simulink model "quad_CAD_asgsm"  (R2024a)
settings: Solver=ode4  StartTime=0.0  StopTime=60  FixedStep=0.01  RelTol=1e-3
undefined symbols (not defined in the file): F, Light, MIL, smiData, X, Y, Z
libraries: sm_lib x221, nesl_utility x22, dspobslib x9, sharedtransform x6, simulink x3, aerolibutil x2, matrix_library x1, sharedutil x1, robotcorelib x1, aerolibwind2 x1
(part 1 of 7)
Description:
  | Adaptive Single-Gain Sliding Mode Controller for a quadrotor modelled in
  | Simscape Multibody
settings Model: Creator=adanm  LastModifiedBy=adanm

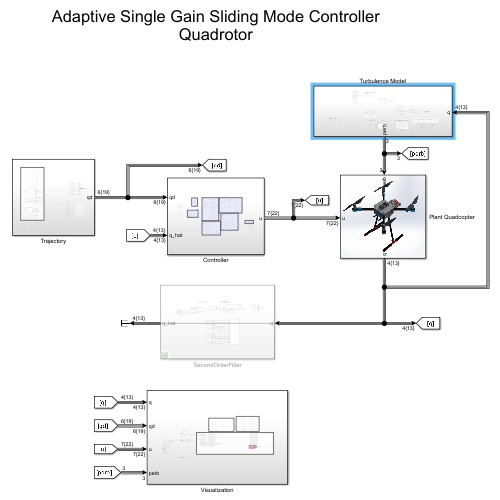
[thumbnail: Simulink's stored preview of the top-level diagram]
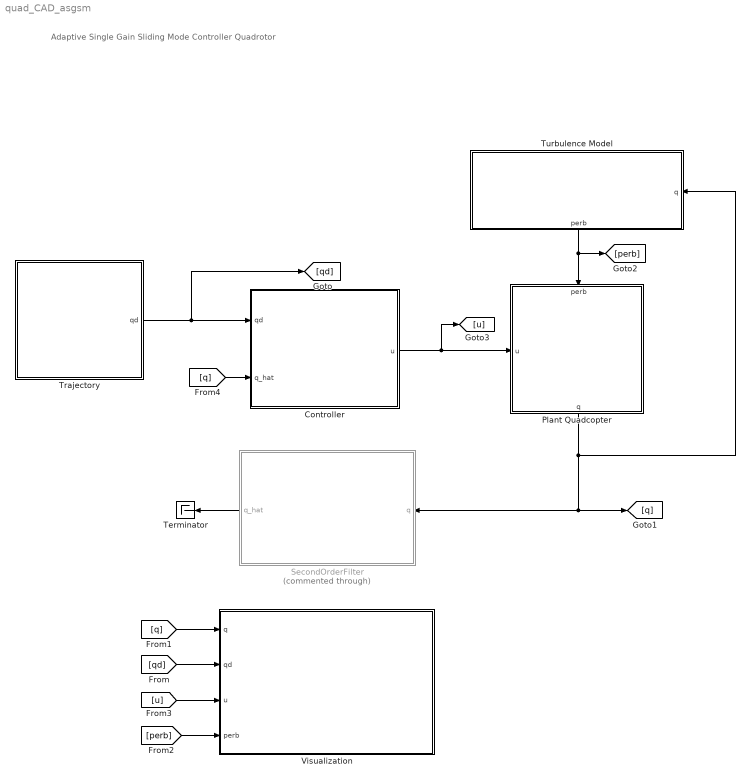
== system quad_CAD_asgsm ==
  note: Adaptive Single Gain Sliding Mode Controller
      | Quadrotor
  Controller : Subsystem
  Plant Quadcopter : Subsystem
      settings: PortSchema="{\"entries\":[{\"content\":{\"sides\":[{\"content\":{\"connectorIds\":[\"In1\"]},\"type\":\"ConnectorPlacement.EquallySpacedRectSide\",\"uuid\":\"f949eb9b-1537-4457-8173-53f8756fded2\"},{\"content\":{\"side\":\"RIGHT\"},\"type\":\"ConnectorPlacement.EquallySpacedRectSide\",\"uuid\":\"4fbfc7d4-94f2-46a4-b9fc-ef834e77a9ed\"},{\"content\":{\"connectorIds\":[\"In2\"],\"side\":\"TOP\"},\"type\":\"ConnectorPlacement.EquallySpacedRectSide\",\"uuid\":\"37f6ffd5-491e-413a-8e1b-4483447938c5\"},{\"content\":{\"connectorIds\":[\"Out1\"],\"side\":\"BOTTOM\"},\"type\":\"ConnectorPlacement.EquallySpacedRectSide\",\"uuid\":\"c1c386c7-2f11-4e96-8840-db3d41072bec\"}]},\"type\":\"ConnectorPlacement.EquallySpacedConnector\",\"uuid\":\"4c6ce227-67e5-4051-af2d-189fa0d9d7e1\"}],\"packageUris\":[\"http://schema.mathworks.com/mf0/Connector/R2020b\"],\"version\":\"1.0\"}"
      mask Display: image('quadRender.png');
  SecondOrderFilter : Subsystem  Commented=through
      settings: PortSchema="{\"entries\":[{\"content\":{\"sides\":[{\"content\":{\"connectorIds\":[\"Out1\"]},\"type\":\"ConnectorPlacement.EquallySpacedRectSide\",\"uuid\":\"b4c8c2cb-3651-490a-ad01-89b97c3933b2\"},{\"content\":{\"connectorIds\":[\"In1\"],\"side\":\"RIGHT\"},\"type\":\"ConnectorPlacement.EquallySpacedRectSide\",\"uuid\":\"f3956ee2-2beb-41a9-b697-53efa6c7f661\"},{\"content\":{\"side\":\"TOP\"},\"type\":\"ConnectorPlacement.EquallySpacedRectSide\",\"uuid\":\"338fc46d-6a44-4c7a-9eb5-4ab91a191b04\"}]},\"type\":\"ConnectorPlacement.EquallySpacedConnector\",\"uuid\":\"d4e003fa-30a1-40f4-b71f-e0999cd1b71b\"}],\"packageUris\":[\"http://schema.mathworks.com/mf0/Connector/R2020b\"],\"version\":\"1.0\"}"
  Terminator : Terminator
  Trajectory : Subsystem
  Turbulence Model : Subsystem
      settings: PortSchema="{\"entries\":[{\"content\":{\"sides\":[{\"content\":{},\"type\":\"ConnectorPlacement.EquallySpacedRectSide\",\"uuid\":\"f78b09a1-2be7-4ada-a431-40e3e9754158\"},{\"content\":{\"connectorIds\":[\"In1\"],\"side\":\"RIGHT\"},\"type\":\"ConnectorPlacement.EquallySpacedRectSide\",\"uuid\":\"90af6136-accc-442b-9679-ef2510f8cfdd\"},{\"content\":{\"side\":\"TOP\"},\"type\":\"ConnectorPlacement.EquallySpacedRectSide\",\"uuid\":\"ed3143b1-02fd-44b4-8f22-c95c41bbcf7f\"},{\"content\":{\"connectorIds\":[\"Out1\"],\"side\":\"BOTTOM\"},\"type\":\"ConnectorPlacement.EquallySpacedRectSide\",\"uuid\":\"715dd93d-905b-40a3-aeb3-61c6c8d9767d\"}]},\"type\":\"ConnectorPlacement.EquallySpacedConnector\",\"uuid\":\"95dc4bc2-a941-4378-8d0a-e3a54b47d1ac\"}],\"packageUris\":[\"http://schema.mathworks.com/mf0/Connector/R2020b\"],\"version\":\"1.0\"}"
  Visualization : Subsystem
  wires:
  Turbulence Model/1(perb) -> [perb], Plant Quadcopter/2(perb)
  Plant Quadcopter/1(q) -> Turbulence Model/1(q), SecondOrderFilter/1(q), [q]
  Trajectory/1(qd) -> [qd], Controller/1(qd)
  SecondOrderFilter/1(q_hat) -> Terminator/1
  Controller/1(u) -> [u], Plant Quadcopter/1(u)
  [qd] -> Visualization/2(qd)
  [q] -> Visualization/1(q)
  [perb] -> Visualization/4(perb)
  [u] -> Visualization/3(u)
  [q] -> Controller/2(q_hat)

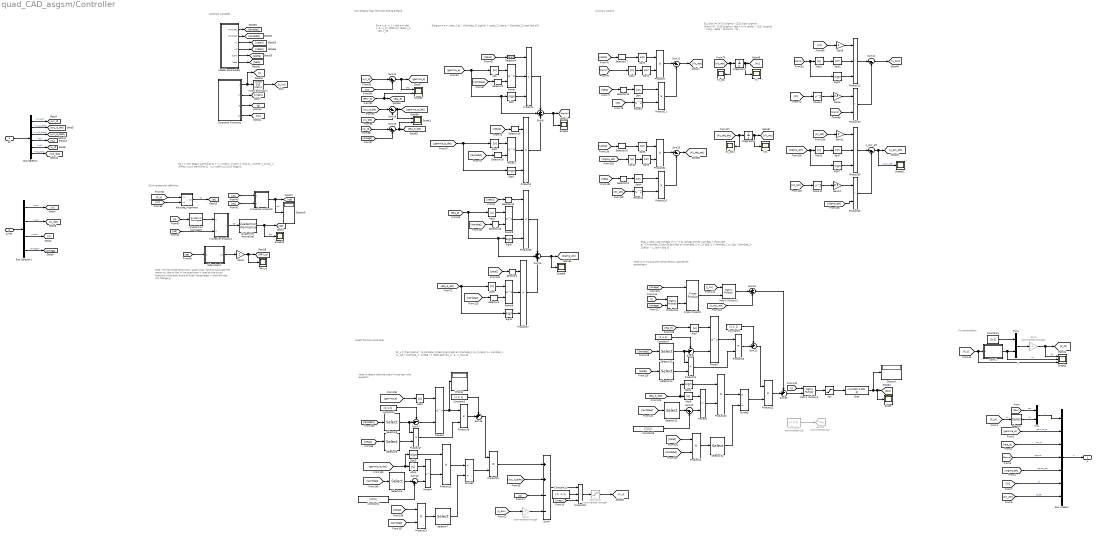
== system quad_CAD_asgsm/Controller ==
  note: $q_t = \pm \Bigg [ \sqrt{\frac{1 + n_u \cdot n_z}{2}} + \frac{n_u \times n_z}{||n_u \times n_z||} \sqrt{\frac{1 - n_u \cdot n_z}{2}} \Bigg ]$
  note: Note: It seems that the mass if missing in
      | the equation.
  note: Note: It is missing the Inertia Tensor outside
      | the parenthesis
  note: $F_u = \frac{|\dot e|^{2-\lambda_2}\text{sign}(\dot e)}{\lambda_2 \xi_2} \Big (1 + \lambda_1 \xi_1|e|^{\lambda_1 - 1}\Big ) + \ddot \gamma_d - g - u_{aux}$
  note: ANSFT Position Controller
  note: $e = x_d - x_1 \\ \dot e = \dot x_d - x_2 \\ \ddot e = \ddot x_d - \dot x_2$
  note: $\sigma = e + \zeta_1 |e| ^{\lambda_1} sign(e) + \zeta_2 | \dot e| ^{\lambda_2} sign(\dot e)$
  note: $u_{aux}=-2K(t) |\sigma|^{1/2} sign (\sigma) - \frac{K(t)^2}{2}\sigma \\ \dot K(t) = \alpha ^{1/2} |\sigma| ^{1/2} - \beta ^{1/2}K(t)^2$
  note: Non-Singular Fast Terminal Sliding Surface
  note: $\tau = \Big [ \dot \omega_d + J^{-1} \omega \times J \omega + \frac{|\dot e|^{2-\lambda_2}\text{sign}(\dot e)}{\lambda_2 \xi_2} \Big (1 + \lambda_1 \xi_1|e|^{\lambda_1 - 1}\Big ) - u_{aux} \Big ]$
  note: Auxiliary Control
  note: Constant variables
  note: Note : For the tilted Hexa-rotor I guess that I
      | have to calculate the vector nz, due to that in the
      | quad-rotor it used as the thrust direction in the body
      | frame of itself. Nonetheless in the FAH that will change ig
  note: Error quaternion definition
  note: Fu manipulation
  qd : Inport
  q_hat : Inport  Port=2
  ASGSM parameters : MATLAB Function  TreatAsAtomicUnit=on
  Abs{,1..11} (12 alike) : Abs  SaturateOnIntegerOverflow=off
  Attitude_Alignment : Subsystem
  Bias : Bias  Bias=[0.002; 0.025; 0]  SaturateOnIntegerOverflow=off
  Bus Creator : BusCreator  Inputs=7
  Bus Selector : BusSelector  OutputSignals=xyz_d,xyz_d_dot,xyz_d_ddot,qz,wd,wd_dot
  Bus Selector1 : BusSelector  OutputSignals=pos,vel,quat,omega
  Constant1 : Constant  Value=[0; 0]
  Constant11 : Constant  Value=[-1; -1; 1]
  Constant{3,5,7,9} (4 alike) : Constant  Value=[1; 1; 1]
  Constant4 : Constant  Value=[2;2;2]
  Constant6 : Constant  Commented=on  Value=[0; 0; 0]
  Constant8 : Constant  Value=[2;2;2]
  Constants Functions : MATLAB Function  TreatAsAtomicUnit=on
  Cross Product1 : matrix_library/Cross Product
  Display : Display
  Display1 : Display
  Display6 : Display
  Divide2 : Product  Inputs=*/
  Divide3 : Product  Inputs=*/
  Gain12 : Gain  Gain=2
  Gain13 : Gain  Gain=0.5
  Gain2 : Gain  Commented=through  Gain=-1
  Gain3 : Gain  Gain=2
  Gain4 : Gain  Commented=through  Gain=-1
  Gain6 : Gain  Gain=2
  Gain8 : Gain  Gain=0.5
  Goto59 : Goto  Commented=on  GotoTag=tau
  Integrator4 : Integrator  InitialCondition=[0;0;0]
  Integrator5 : Integrator  InitialCondition=[0;0;0]
  Invert 3x3 Matrix : aerolibutil/Invert  3x3 Matrix
  Kronecker product3 : Subsystem
  Kronecker product4 : Subsystem
  Kt : Scope
  Kt1 : Scope
  Kt_dot : Scope
  Kt_dot1 : Scope
  Matrix Multiply2 : Product  Multiplication=Matrix(*)
  Matrix Multiply5 : Product  Multiplication=Matrix(*)
  Mux : Mux  Inputs=2
  Mux1 : Mux  Inputs=2
  PRV_e : Scope
  Power{,1,4..9} (8 alike) : Math  Operator=pow
  Power{2..3,10..11} (4 alike) : Math  Operator=square
  Product{9..11,13..17,20..24,28..29,31} (16 alike) : Product
  Product{4,8,12,25..27,30} (7 alike) : Product  Inputs=3
  Product19 : Product  Multiplication=Matrix(*)
  Quaternion Conjugate : aerolibutil/Quaternion Conjugate
  Quaternion Normalize1 : sharedutil/Quaternion Normalize  aMode=aMode
  Saturation : Saturate  Commented=through  UpperLimit=4*10  LowerLimit=0
  Scope{,8..11} (5 alike) : Scope
  Scope1 : Scope  NumInputPorts=2
  Scope2 : Scope  NumInputPorts=3
  Scope3 : Scope  NumInputPorts=2
  Selector : Selector  InputPortWidth=3  IndexOptions=Index vector (dialog)  Indices=[3]  OutputSizes=1
  Selector{1,3,10..14,18,20..21} (10 alike) : Selector  InputPortWidth=6  IndexOptions=Index vector (dialog)  Indices=[4:6]  OutputSizes=1
  Selector{4..9,15..17,19} (10 alike) : Selector  InputPortWidth=6  IndexOptions=Index vector (dialog)  Indices=[1:3]  OutputSizes=1
  Sign{,1..7} (8 alike) : Signum
  Sqrt{,1..7} (8 alike) : Sqrt
  Subsystem1 : Subsystem
  Sum10 : Sum  Inputs=|-+
  Sum{11,14..16,25} (5 alike) : Sum  Inputs=|+-
  Sum12 : Sum  Inputs=|--
  Sum17 : Sum  Inputs=-+|
  Sum18 : Sum  Inputs=++|
  Sum19 : Sum  Inputs=++-
  Sum20 : Sum  Inputs=|-+
  Sum21 : Sum  Inputs=-+|
  Sum22 : Sum  Inputs=++|
  Sum23 : Sum  Inputs=++|
  Sum24 : Sum  Inputs=+++
  Sum6 : Sum  Inputs=++--
  Sum9 : Sum  Inputs=+++
  norm1 : MATLAB Function  TreatAsAtomicUnit=on
  tau : Saturate
  u_aux_att : Sum  Inputs=|--
  u : Outport
  wires:
  Sqrt5/1 -> Product31/1
  Sum14/1 -> Scope3/1, [gamma_e]  "des"
  Product28/1 -> u_aux_att/2
  u_aux_att/1 -> Scope11/1, [u_aux_att]  "u_aux_att"
  Sum12/1 -> [u_aux]
  Product29/1 -> Sum25/2
  Integrator4/1 -> Kt/1, [Kt]
  Selector19/1 -> Sqrt/1
  [J] -> Matrix Multiply5/1
  [sigma_att] -> Product28/2
  [g] -> Sum6/3
  Product22/1 -> Sum23/2
  Sum10/1 -> Power4/2
  Cross Product1/1 -> Matrix Multiply2/2
  Sqrt3/1 -> Product12/2
  Abs7/1 -> Power7/1
  Sum25/1 -> [Kt_dot_att]
  Selector20/1 -> Sqrt5/1
  [Kt_att] -> Gain12/1
  [lambda2] -> Selector3/1
  Selector18/1 -> Power8/2
  [omega] -> Cross Product1/1
  Sqrt7/1 -> Product30/2
  [xyz_d_ddot] -> Sum6/2
  Sum24/1 -> Scope8/1, [sigma_att]
  Product27/1 -> Sum24/3
  Selector7/1 -> Divide2/2
  Power10/1 -> Product29/2
  Sign6/1 -> Product27/3
  Sign/1 -> Product4/3
  Sum19/1 -> Sum23/1
  Abs11/1 -> Sqrt7/1
  [eta_e_dot] -> Abs9/1, Sign6/1
  Sum20/1 -> Power6/2
  Selector5/1 -> Power/2
  [gamma_e] -> Abs5/1
  [PRV_e] -> Scope3/2, [eta_e]
  [gamma_e] -> Sum9/2, Sign/1, Abs/1
  [eta_e] -> Sum24/2, Sign5/1, Abs8/1
  Power8/1 -> Product26/2
  Abs8/1 -> Power8/1
  Product26/1 -> Sum24/1
  Abs5/1 -> Power5/1
  Constant8/1 -> Sum20/2
  Selector3/1 -> Power9/2
  Selector17/1 -> Sqrt1/1
  Sum17/1 -> Power5/2
  Selector16/1 -> Power1/2
  Abs6/1 -> Power6/1
  [Kt_dot_att] -> Kt_dot1/1, Integrator5/1
  Constant9/1 -> Sum22/1
  [Kt_att] -> Power10/1
  Constant5/1 -> Sum18/1
  Sign7/1 -> Product30/3
  Selector9/1 -> Product17/2
  Sqrt4/1 -> Product29/1
  Constant11/1 -> Product25/2
  Abs1/1 -> Power1/1
  Product25/1 -> Saturation/1
  Selector21/1 -> Sqrt4/1
  Sum6/1 -> Product25/1
  [lambda1] -> Selector13/1
  Selector13/1 -> Product24/1, Sum21/2
  [Kt] -> Power2/1
  Power4/1 -> Product13/2
  Power7/1 -> Product23/1
  Selector12/1 -> Divide3/2
  [lambda2] -> Selector11/1
  Constant3/1 -> Sum17/1
  Sum11/1 -> [Kt_dot]
  Sign4/1 -> Product20/1
  Product23/1 -> Sum22/2
  [lambda2] -> Product21/2
  Product21/1 -> Selector12/1
  Constant7/1 -> Sum21/1
  Power6/1 -> Product20/2
  Selector14/1 -> Product24/2
  [zeta2] -> Product21/1
  Power1/1 -> Product8/2
  [J_inv] -> Matrix Multiply2/1
  Product15/1 -> Sum6/1
  Matrix Multiply5/1 -> tau/1
  Product17/1 -> Product16/2
  Product16/1 -> Sum18/2
  Product20/1 -> Divide3/1
  Power9/1 -> Product27/2
  [w_d] -> Sum16/1
  Abs3/1 -> Sqrt3/1
  Selector8/1 -> Product17/1, Sum17/2
  Gain4/1 -> Sum6/4
  Product14/1 -> Selector7/1
  Divide2/1 -> Product15/2
  Power3/1 -> Gain8/1
  [lambda2] -> Product14/2
  [alpha] -> Selector20/1
  Product13/1 -> Divide2/1
  Abs4/1 -> Power4/1
  Abs2/1 -> Sqrt2/1
  [Kt_att] -> Power11/1
  [gamma_e_dot] -> Sign3/1, Abs4/1
  [xi] -> Sum14/2
  [lambda1] -> Selector5/1
  [sigma] -> Product10/2
  [xyz_d_dot] -> Sum15/1
  Product30/1 -> u_aux_att/1
  [lambda2] -> Selector6/1
  [zeta2] -> Selector1/1
  [xyz_d] -> Sum14/1
  [u_aux] -> Gain4/1
  Selector6/1 -> Sum10/1
  Product11/1 -> Sum11/2
  Sqrt1/1 -> Product9/1
  [zeta1] -> Selector9/1
  [xi_dot] -> Sum15/2
  Selector1/1 -> Product27/1
  [beta] -> Selector19/1
  [gamma_e_dot] -> Sign1/1, Abs1/1
  Product4/1 -> Sum9/1
  [lambda2] -> Selector16/1
  tau/1 -> Bias/1
  [zeta2] -> Selector15/1
  [Kt_dot] -> Kt_dot/1, Integrator4/1
  [zeta1] -> Selector4/1
  Sum16/1 -> Scope1/2, [eta_e_dot]
  Product12/1 -> Sum12/1
  [alpha] -> Selector17/1
  [sigma_att] -> Abs10/1
  Sign1/1 -> Product8/3
  Product8/1 -> Sum9/3
  [sigma_att] -> Abs11/1, Sign7/1
  [u_aux_att] -> Sum19/3
  [omega] -> Sum16/2
  Power2/1 -> Product11/2
  Power11/1 -> Gain13/1
  Abs10/1 -> Sqrt6/1
  Abs9/1 -> Power9/1
  Integrator5/1 -> Kt1/1, [Kt_att]
  Sign3/1 -> Product13/1
  Constant6/1 -> Goto59/1
  [eta_e] -> Abs7/1
  Product10/1 -> Sum12/2
  Gain6/1 -> Product12/1
  Sum21/1 -> Power7/2
  Gain12/1 -> Product30/1
  Selector10/1 -> Product26/1
  [eta_e_dot] -> Sign4/1, Abs6/1
  [zeta2] -> Product14/1
  Product9/1 -> Sum11/1
  [lambda1] -> Selector8/1
  Selector11/1 -> Sum20/1
  [zeta1] -> Selector14/1
  Sign5/1 -> Product26/3
  Sqrt/1 -> Product11/1
  Gain13/1 -> Product28/1
  Product19/1 -> Cross Product1/2
  [omega] -> Product19/2
  Sign2/1 -> Product12/3
  Matrix Multiply2/1 -> Sum19/2
  [Kt] -> Power3/1
  Abs/1 -> Power/1
  [sigma] -> Sign2/1, Abs3/1
  [lambda1] -> Selector18/1
  Product24/1 -> Product23/2
  Sum9/1 -> Scope9/1, [sigma]
  [sigma] -> Abs2/1
  [beta] -> Selector21/1
  Gain8/1 -> Product10/1
  Sum23/1 -> Matrix Multiply5/2
  Sum18/1 -> Product15/1
  Product31/1 -> Sum25/1
  Constant4/1 -> Sum10/2
  Sqrt2/1 -> Product9/2
  Sum22/1 -> Product22/1
  Selector15/1 -> Product8/1
  Divide3/1 -> Product22/2
  Sqrt6/1 -> Product31/2
  Power5/1 -> Display/1, Product16/1
  [zeta1] -> Selector10/1
  Selector4/1 -> Product4/1
  [J] -> Product19/1
  Power/1 -> Product4/2
  [Kt] -> Gain6/1
  ASGSM parameters/1(lambda1) -> [lambda1]
  ASGSM parameters/2(lambda2) -> [lambda2]
  ASGSM parameters/3(xi1) -> [zeta1]
  ASGSM parameters/5(alpha) -> [alpha]
  Constants Functions/1(J) -> [J], Invert 3x3 Matrix/1
  ASGSM parameters/6(beta) -> [beta]
  ASGSM parameters/4(xi2) -> [zeta2]
  Constants Functions/3(g) -> [g]
  Constants Functions/4(nz) -> [nz]
  Invert 3x3 Matrix/1 -> [J_inv]
  Constants Functions/2(m) -> [mass]
  [q] -> Quaternion Conjugate/1
  Attitude_Alignment/1(qt) -> [qt]  "qt"
  [F_u] -> Attitude_Alignment/1(nu)
  Kronecker product4/1(r) -> Quaternion Normalize1/1  "qe"
  Kronecker product3/1(r) -> Display6/1, [qd]  "qd"
  Subsystem1/1(lnq) -> Gain3/1
  [nz] -> Attitude_Alignment/2(nz)
  [qe] -> Subsystem1/1(q)
  [qz] -> Kronecker product3/2(p)
  Quaternion Normalize1/1 -> Scope10/1, [qe]  "qe"
  Gain3/1 -> PRV_e/1, [PRV_e]
  [qt] -> Kronecker product3/1(q)
  Quaternion Conjugate/1 -> Kronecker product4/1(q)
  [qd] -> Kronecker product4/2(p)
  Gain2/1 -> [F_th], Scope2/1  "fth"
  Mux1/1 -> Gain2/1
  norm1/1(y) -> Mux1/2, Scope2/2  "nu"
  Constant1/1 -> Mux1/1
  [F_u] -> norm1/1(u), Scope2/3  "fu"
  [tau] -> Mux/1  "tau"
  [F_th] -> Selector/1  "fu"
  Bus Creator/1 -> u/1  "u"
  qd/1 -> Bus Selector/1
  q_hat/1 -> Bus Selector1/1
  Bus Selector1/3 -> [q]  "<quat>"
  Bus Selector/1 -> [xyz_d]  "<xyz_d>"
  Bus Selector/2 -> [xyz_d_dot]  "<xyz_d_dot>"
  Bus Selector1/2 -> [xi_dot]  "<vel>"
  Bus Selector1/4 -> [omega]  "<omega>"
  Bus Selector1/1 -> [xi]  "<pos>"
  Bus Selector/3 -> [xyz_d_ddot]  "<xyz_d_ddot>"
  Bus Selector/5 -> [w_d]  "<wd>"
  Selector/1 -> Mux/2  "fu"
  Bus Selector/4 -> [qz]  "<qz>"
  Mux/1 -> Bus Creator/1  "u"
  [gamma_e] -> Bus Creator/2  "gamma_e"
  [eta_e] -> Bus Creator/3  "prv_e"
  [sigma] -> Bus Creator/4  "sigma"
  [sigma_att] -> Bus Creator/5  "sigma_att"
  [Kt] -> Bus Creator/6  "kt"
  [Kt_att] -> Bus Creator/7  "kt_att"
  [mass] -> Product25/3
  Sum15/1 -> Scope1/1, [gamma_e_dot]
  Bias/1 -> Display1/1, Scope/1, [tau]
  Bus Selector/6 -> [wd_dot]  "<wd_dot>"
  Saturation/1 -> [F_u]
